simulink model "tisch"  (Simulink 8.2)
settings: Solver=ode45  StartTime=0.0  StopTime=10.0  RelTol=1e-3
settings Model: Creator=abx968  LastModifiedBy=abx968
settings DataIOCC: SignalLoggingSaveFormat=Dataset
settings OptimizationCC: ExpressionDepthLimit=128
settings DebuggingCC: FcnCallInpInsideContextMsg=EnableAllAsError  StateNameClashWarn=none
settings GRTTargetCC: CombineOutputUpdateFcns=on  GRTInterface=off

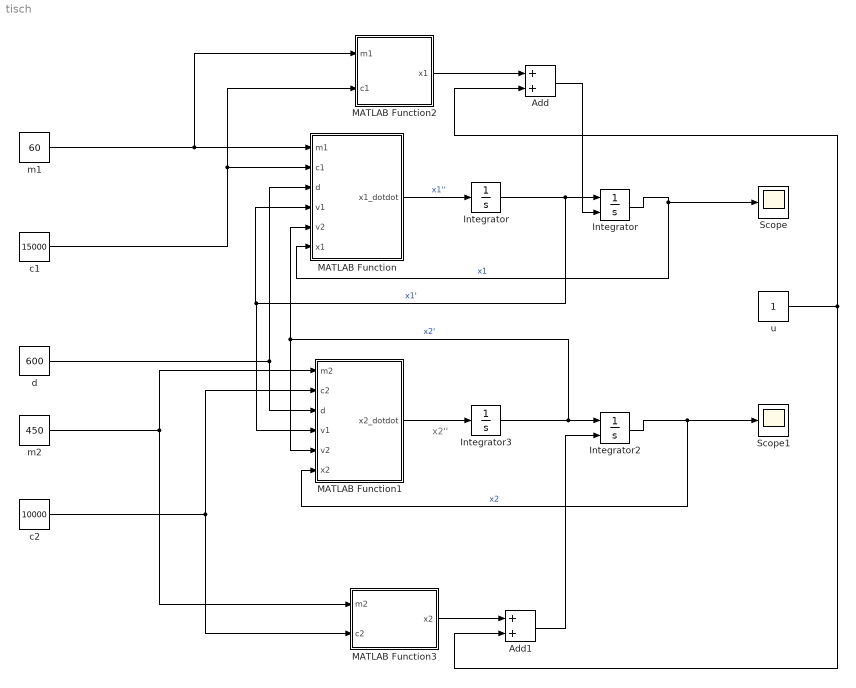
== system tisch ==
  note: x2''
  Add : Sum
  Add1 : Sum
  Integrator : Integrator  InitialConditionSource=external
  "Integrator " : Integrator
  Integrator2 : Integrator  InitialConditionSource=external
  Integrator3 : Integrator
  MATLAB Function : MATLAB Function  TreatAsAtomicUnit=on
  MATLAB Function1 : MATLAB Function  TreatAsAtomicUnit=on
  MATLAB Function2 : MATLAB Function  TreatAsAtomicUnit=on
  MATLAB Function3 : MATLAB Function  TreatAsAtomicUnit=on
  Scope : Scope
  Scope1 : Scope
  c1 : Constant  Value=15000
  c2 : Constant  Value=10000
  d : Constant  Value=600
  m1 : Constant  Value=60
  m2 : Constant  Value=450
  u : Constant
  wires:
  Integrator/1 -> MATLAB Function/6(x1), Scope/1  "x1"
  Integrator2/1 -> MATLAB Function1/6(x2), Scope1/1  "x2"
  Integrator3/1 -> MATLAB Function/5(v2), MATLAB Function1/5(v2), Integrator2/1  "x2'"
  MATLAB Function/1(x1_dotdot) -> "Integrator "/1  "x1''"
  "Integrator "/1 -> MATLAB Function1/4(v1), MATLAB Function/4(v1), Integrator/1  "x1'"
  MATLAB Function1/1(x2_dotdot) -> Integrator3/1
  m1/1 -> MATLAB Function2/1(m1), MATLAB Function/1(m1)
  c1/1 -> MATLAB Function2/2(c1), MATLAB Function/2(c1)
  d/1 -> MATLAB Function/3(d), MATLAB Function1/3(d)
  m2/1 -> MATLAB Function1/1(m2), MATLAB Function3/1(m2)
  c2/1 -> MATLAB Function1/2(c2), MATLAB Function3/2(c2)
  MATLAB Function3/1(x2) -> Add1/1
  MATLAB Function2/1(x1) -> Add/1
  u/1 -> Add1/2, Add/2
  Add1/1 -> Integrator2/2
  Add/1 -> Integrator/2

== matlab function MATLAB Function1 ==
  data: m2 input double; x2_dotdot output double; c2 input double; d input double; v1 input double; v2 input double; x2 input double
function x2_dotdot = fcnx2(m2,c2,d,v1,v2,x2)
g = 9.81;
x2_dotdot = (2*c2*(-x2) - m2*g - (v2-v1)*d) / m2;

== matlab function MATLAB Function ==
  data: m1 input double; x1_dotdot output double; c1 input double; d input double; v1 input double; v2 input double; x1 input double
function x1_dotdot = fcnx1(m1,c1,d,v1,v2,x1)
g = 9.81;
x1_dotdot = (2*c1*(-x1) - m1*g + (v2-v1)*d) / m1;

== matlab function MATLAB Function2 ==
  data: m1 input double; x1 output double; c1 input double
function x1 = fcnx1start(m1,c1)
g = 9.81;
x1 = (-m1*g)/(2*c1);

== matlab function MATLAB Function3 ==
  data: m2 input double; x2 output double; c2 input double
function x2 = fcnx2start(m2,c2)
g = 9.81;
x2 = (-m2*g)/(2*c2);
